simulink model "Position_State_Feedback_Motor"  (R2021b)
settings: Solver=FixedStepAuto  StartTime=0.0  StopTime=15  RelTol=1e-3  EnableMultiTasking=on
undefined symbols (not defined in the file): Ts
libraries: mbedblockslib x3, stm_qeplib x1
settings Model: ExtModeTrigDuration=10  Creator=UTENTE  LastModifiedBy=UTENTE
settings OptimizationCC: EnhancedBackFolding=on  PassReuseOutputArgsAs=Individual arguments  ZeroExternalMemoryAtStartup=off  ZeroInternalMemoryAtStartup=off  MaxStackSize=64  OptimizeBlockOrder=speed  DifferentSizesBufferReuse=on  OptimizationCustomize=off  EfficientTunableParamExpr=on
settings DebuggingCC: ParameterTunabilityLossMsg=error
settings HardwareCC: ProdBitPerPointer=32  ProdBitPerSizeT=32  ProdBitPerPtrDiffT=32  ProdLargestAtomicInteger=Long  ProdLargestAtomicFloat=Double  ProdWordSize=32  ProdLongLongMode=on  ProdHWDeviceType=ARM Compatible->ARM Cortex
settings SFSimCC: MATLABDynamicMemAlloc=off
settings RTWCC: Description=Embedded Coder  SystemTargetFile=ert.tlc  HardwareBoard=STM32 Nucleo F401RE  TemplateMakefile=ert_default_tmf  Toolchain=GNU Tools for ARM Embedded Processors  PortableWordSizes=on
settings CodeAppCC: ForceParamTrailComments=on  IgnoreCustomStorageClasses=off  OperatorAnnotations=on  SimulinkDataObjDesc=on  SFDataObjDesc=on  InsertBlockDesc=on
settings ERTTargetCC: ExtModeTransport=3  ExtModeStaticAlloc=on  ExtModeStaticAllocSize=2000  ExtModeMexFile=ext_xcp  ExtModeIntrfLevel=Level2 - Open

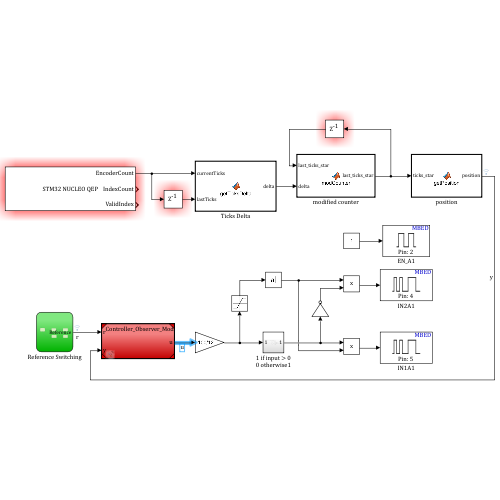
[thumbnail: Simulink's stored preview of the top-level diagram]
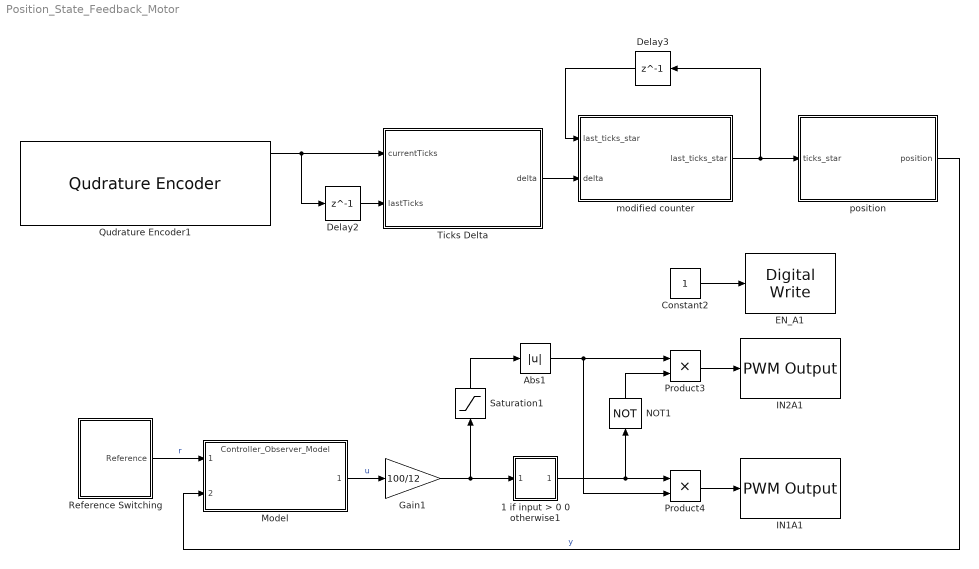
== system Position_State_Feedback_Motor ==
  1 if input > 0 0 otherwise1 : Subsystem
  Abs1 : Abs
  Constant2 : Constant
  Delay2 : Delay  DelayLength=1  InitialCondition=0  SampleTime=Ts
  Delay3 : Delay  DelayLength=1  InitialCondition=0  SampleTime=Ts
  EN_A1 : mbedblockslib/Digital Write  Pin=2  Direction=output
      settings: SourceProductBaseCode=MICROBIT,NUCLEO,STMICRODIS
  Gain1 : Gain  Gain=100/12
  IN1A1 : mbedblockslib/PWM Output  Pin=5  EnableInputFrequency=off  InitialFrequency=pwmFreq  InitialDutyCycle=0  NotificationType=None
      settings: SourceProductBaseCode=MICROBIT,NUCLEO,STMICRODIS
  IN2A1 : mbedblockslib/PWM Output  Pin=4  EnableInputFrequency=off  InitialFrequency=pwmFreq  InitialDutyCycle=0  NotificationType=None
      settings: SourceProductBaseCode=MICROBIT,NUCLEO,STMICRODIS
  Model : ModelReference  ModelNameDialog=Controller_Observer_Model.slx  SimulationMode=Normal  ModelReferenceVersion=1.47
  NOT1 : Logic  Operator=NOT  IconShape=distinctive  AllPortsSameDT=off  OutDataTypeStr=boolean
  Product3 : Product
  Product4 : Product
  Qudrature Encoder1 : stm_qeplib/Qudrature Encoder  SampleTime=Ts
  Reference Switching : Stateflow chart  TreatAsAtomicUnit=on
  Saturation1 : Saturate  UpperLimit=100  LowerLimit=-100
  Ticks Delta : MATLAB Function  TreatAsAtomicUnit=on
  modified counter : MATLAB Function  TreatAsAtomicUnit=on
  position : MATLAB Function  TreatAsAtomicUnit=on
  wires:
  position/1(position) -> Model/2  "y"
  Model/1 -> Gain1/1  "u"
  modified counter/1(last_ticks_star) -> Delay3/1, position/1(ticks_star)
  Product4/1 -> IN1A1/1
  Delay3/1 -> modified counter/1("last_ticks_star ")
  1 if input > 0 0 otherwise1/1(Out1) -> Product4/1, NOT1/1
  Gain1/1 -> Saturation1/1, 1 if input > 0 0 otherwise1/1(In1)
  Abs1/1 -> Product4/2, Product3/1
  Delay2/1 -> Ticks Delta/2(lastTicks)
  Constant2/1 -> EN_A1/1
  Qudrature Encoder1/1 -> Ticks Delta/1(currentTicks), Delay2/1
  NOT1/1 -> Product3/2
  Ticks Delta/1(delta) -> modified counter/2(delta)
  Saturation1/1 -> Abs1/1
  Product3/1 -> IN2A1/1
  Reference Switching/1(Reference) -> Model/1  "r"

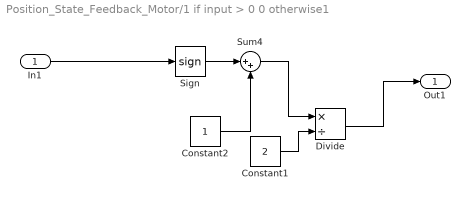
== system Position_State_Feedback_Motor/1 if input > 0 0 otherwise1 ==
  In1 : Inport
  Constant1 : Constant  Value=2
  Constant2 : Constant
  Divide : Product  Inputs=*/
  Sign : Signum
  Sum4 : Sum  Inputs=|++
  Out1 : Outport
  wires:
  Sum4/1 -> Divide/1
  Constant2/1 -> Sum4/2
  Sign/1 -> Sum4/1
  Divide/1 -> Out1/1
  In1/1 -> Sign/1
  Constant1/1 -> Divide/2

== stateflow chart Position_State_Feedback_Motor/Reference Switching ==
  state S1
    Reference=0;
  state S2
    Reference=-pi;
  state S3
    Reference=pi;
  state s6
    Reference=0;
  state s5
    Reference=2*pi;
  (default) -> S1
  S1 -> S2 : after(2,sec)
  S2 -> S3 : after(2,sec)
  S3 -> s5 : after(2,sec)
  s6 -> S1 : after(2,sec)
  s5 -> s6 : after(2,sec)
  data: Reference output

== matlab function Position_State_Feedback_Motor/modified counter ==
  data: last_ticks_star input; last_ticks_star output; delta input
function last_ticks_star = modCounter(last_ticks_star,delta)
     sum = last_ticks_star+delta;
	 last_ticks_star = sign(sum)*mod(abs(sum),89796);

end

== matlab function Position_State_Feedback_Motor/position ==
  data: ticks_star input; position output
function position = getPosition(ticks_star)

ticks_star = double(ticks_star);

position = 2*pi*ticks_star/(3591.84);


end

== matlab function Position_State_Feedback_Motor/Ticks Delta ==
  data: currentTicks input; delta output; lastTicks input; Ts parameter
function delta = getTicksDelta(currentTicks, lastTicks, Ts)
    currentTicks = double(currentTicks);
    lastTicks = double(lastTicks);
  
    if abs(currentTicks-lastTicks) <= ceil(8400*Ts) 
	     delta = currentTicks-lastTicks;
    else
    if lastTicks>currentTicks
	     delta = currentTicks+2^16-1-lastTicks;
    else
	     delta = currentTicks-2^16+1-lastTicks;
	    end
end

end
